simulink model "ansiBPF"  (R2018a)
settings: Solver=VariableStepAuto  StartTime=0.0  StopTime=0.001  RelTol=1e-3
undefined symbols (not defined in the file): fdesignblkfcn, G1, G10, G11, G12, G13, G14, G15, G16, G17, G18, G19, G2, G20, G21, G22, G23, G24, G25, G26, G3, G4, G5, G6, G7, G8, G9, gcbh, get, T
libraries: dspsrcs4 x1, dspxfrm3 x1, dspobslib x1
(part 2 of 8)

== system ansiBPF/Filter Bank /Filter 1/Bandpass Filter ==
  In : Inport
  Generated Filter Block : DiscreteFir  Tag=BlockMethodSubSystem  Coefficients=[0.0499507052705291318 0.000322270032915632448 0.000320188963324847956 0.000323977422964133151 0.000321713773073391111 0.000325363631786397078 0.000322903780407593076 0.000326435292404190028 0.000323726665637299603 0.000327135403143973057 0.000324164311384914105 0.000327508044235636268 0.000324274377688199664 0.000327562416867693297 0.000323957726949763232 0.000327232187704450399 0.000323344949635380897 0.000326624522215911107 0.000322307254760139392 0.00032580787553647487 0.000320960780481276359 0.000324697279934548508 0.000319257227297288124 0.000323532322174875826 0.000317320055412668978 0.000322525688887117048 0.000315188666134388798 0.000322272842734003641 0.000313133698767870767 0.000324938293286081007 0.000311846130644410772 0.000347911651016281258 0.000403441686760817907 0.000297983621868963587 0.000325553998969463972 0.000314801796637866754 0.000322376414307447051 0.000316225568461547747 0.000319627270835727822 0.000315367721629143639 0.000316827696566097548 0.000313550600974511317 0.000313841748774321551 0.000311178641818180696 0.000310645179700694935 0.000308339589890846433 0.000307082402857562927 0.00030506389195534921 0.000303289042348015166 0.000301392710367551664 0.000299107424724176681 0.000297449923396902593 0.000294574508449678548 0.000293085034438766946 0.000289703193611834018 0.000288524166281404896 0.000284574756131985857 0.000283864586364604053 0.000279247312497059091 0.00027950989385441366 0.000274059887801314614 0.000276778817366210507 0.000269800258802989237 0.000284929243345160492 0.000283667983013746879 0.000256341854324833524 0.000266246888784617503 0.000258441820358657945 0.000259919445659265625 0.000254271235270379003 0.000253863599798776569 0.000249074864716378533 0.000247701743744928619 0.000243346757243663713 0.00024135746450751195 0.000237267929251366465 0.000234794357897953599 0.00023080360466084252 0.000227870792300621783 0.000224002787101546024 0.000220716617566540094 0.000216796407569049151 0.000213204269357036554 0.000209323511238944897 0.000205277865080490173 0.000201412148869970322 0.000197030453623327732 0.000193257883064897366 0.000188493476993681667 0.000184903345259595614 0.000179758531360253672 0.00017669703079523582 0.0001712125296252561 0.000169594176652715855 0.000163669815242406888 0.000169209483617797527 0.000158691626351559895 0.000147141133803010521 0.000148689909581561111 0.000141419334482159468 0.000139026139903162128 0.000132817354956990422 0.000129471877618246014 0.000123647868192018444 0.000119769347168019225 0.000114128631332419424 0.000109899614122812946 0.000104355797795147015 9.98123926371075184e-05 9.42446037635563634e-05 8.94063108954827563e-05 8.38853496698552595e-05 7.87737989141462636e-05 7.31343128585705744e-05 6.78500081840607247e-05 6.21201361671771922e-05 5.64867904529115343e-05 5.07067815823427086e-05 4.48484184389351008e-05 3.9038446040410134e-05 3.29178180392793651e-05 2.71387403106747555e-05 2.08276072283989303e-05 1.53374637248327835e-05 8.9858584085083406e-06 4.34843225694638722e-06 -1.84041404762174528e-06 -2.61999962832273039e-06 -1.53795105204806869e-05 -2.23167825954521411e-05 -2.60238776460634881e-05 -3.35303089579822711e-05 -3.88675007855140896e-05 -4.59356687316810194e-05 -5.1714332151380571e-05 -5.86588787380864666e-05 -6.47087092550114023e-05 -7.15961180700431057e-05 -7.78259186883305221e-05 -8.47019799255221972e-05 -9.11297010712597624e-05 -9.80755165498401588e-05 -0.000104664659704481594 -0.000111595264430823393 -0.000118399687148734549 -0.000125440312275471613 -0.000132323624602139243 -0.000139529297481968365 -0.000146653678106061435 -0.000153918626685325337 -0.00016118239140813594 -0.000168535424938574872 -0.00017596314172899701 -0.000183348683518542473 -0.000190821075256901413 -0.000198039321408629101 -0.000205357267343941993 -0.00021208883464483543 -0.000218927092046725141 -0.000224088820977669527 -0.000236938143622294708 -0.000242792916361279367 -0.000249855402636313883 -0.000257730566739408781 -0.000265167623686717198 ...(+30966 chars)]  InputProcessing=Columns as channels (frame based)
  Out : Outport
  wires:
  In/1 -> Generated Filter Block/1
  Generated Filter Block/1 -> Out/1

== system ansiBPF/Filter Bank /Filter 10/Bandpass Filter ==
  In : Inport
  Generated Filter Block : DiscreteFir  Tag=BlockMethodSubSystem  Coefficients=[-0.00530401889529867176 -0.000762503662223860588 -0.000809597041362384662 -0.00085423713825715918 -0.000894486120251178156 -0.00093107548534541811 -0.000962288947070095253 -0.000989049435271363749 -0.00100934406038991867 -0.00102410104453707035 -0.00103149455372060885 -0.00103223687206899358 -0.00102448142749090036 -0.00100884844553548558 -0.000983515907192630172 -0.000949243642068295455 -0.000904319526077239279 -0.000849733841231411547 -0.000784037714204466958 -0.000708543736320957069 -0.000622127019485820172 -0.000526256294042048967 -0.000419644908513648965 -0.000303518853045686623 -0.000175943274000202999 -3.82552865238885645e-05 0.000111501683883899355 0.000270568478960216054 0.000438231571149218875 0.000609275407521666962 0.000787476786344833385 0.000986628487263300916 0.00117728994401449503 0.00137958302728576087 0.00158529722033642147 0.0017943167270931266 0.00200587609221354254 0.00221835053007343307 0.00243145506573108237 0.00264299880656624275 0.00285260919893783093 0.00305799897700812732 0.00325867434990166367 0.00345224276972189072 0.0036381525181242518 0.00381397827273103913 0.00397934470676978343 0.00413193515136546681 0.00427148440753266634 0.00439563199552642052 0.00450393141663923621 0.00459396169417253079 0.00466534335796109194 0.00471596849442543903 0.0047460829476344028 0.00475372894601983932 0.00473965666642539932 0.00470092950151681632 0.0046374213913586192 0.00454736880213954271 0.00443390292271470497 0.00429527524807777391 0.00412717617392089915 0.00393592745618333989 0.003717549896623055 0.00347337100296327616 0.00320396823719764842 0.00290931484653729911 0.00259092019299267135 0.00224862188594879839 0.00188446325206646933 0.00149863620390504608 0.00109346550765449489 0.000669391686506665292 0.00022891711714851542 -0.000227267110878131347 -0.000696281888405515911 -0.00117708989182640079 -0.00166649774040128159 -0.00216330051213994802 -0.00266433060412914636 -0.00316826631716930675 -0.00367190191018134608 -0.00417353296082717973 -0.00466960689996043232 -0.00515833134124038788 -0.00563589955200152586 -0.00610175871945096548 -0.00655196129802019904 -0.00698462243668052964 -0.00739547327021302433 -0.0077846372227648522 -0.00814879846851517507 -0.00848416723132251402 -0.00879058807074419371 -0.00906503847972718775 -0.00930543067975272975 -0.00951046410337792227 -0.00967774427538462163 -0.00980673524036465051 -0.00989502796839583469 -0.00994245078282056383 -0.00994696268261321265 -0.00990885487066216382 -0.00982662150586692019 -0.00970098126763126525 -0.00953077187132917066 -0.00931705690973690104 -0.00905904662331406124 -0.00875829750638353402 -0.00841465404343268338 -0.00803011316082513117 -0.0076051069870370679 -0.00714173367553548599 -0.00664085703672448978 -0.00610487290695389644 -0.00553514255694706123 -0.00493553731689033368 -0.00430658657183950657 -0.00365199467779552195 -0.00297358801683265646 -0.00227607748273341579 -0.00156041508850677472 -0.000830591097045980942 -9.02778463345356327e-05 0.000657701321223840181 0.00141012165207445592 0.00216301715968920906 0.00291355772225113541 0.00365735681289422162 0.00439198914739929048 0.00511302399646780363 0.00581814101116282911 0.00650291241124247802 0.00716505438872799393 0.0078003378917738328 0.00840677071557788605 0.00898045304128435376 0.00951971831009208735 0.0100209022066045667 0.0104825303066184029 0.0109013417773679965 0.0112761257041957674 0.0116044375129104368 0.0118852844436046212 0.012116974638974664 0.0122984597861088285 0.0124280462570238032 0.0125069270388523026 0.0125329151884100362 0.0125069270388523026 0.0124280462570238032 0.0122984597861088285 0.012116974638974664 0.0118852844436046212 0.0116044375129104368 0.0112761257041957674 0.0109013417773679965 0.0104825303066184029 0.0100209022066045667 0.00951971831009208735 0.00898045304128435376 0.00840677071557788605 0.0078003378917738328 0.00716505438872799393 0.00650291241124247802 0.00581814101116282911 0.00511302399646780363 0.00439198914739929048 0.00365735681289422162 ...(+3064 chars)]  InputProcessing=Columns as channels (frame based)
  Out : Outport
  wires:
  In/1 -> Generated Filter Block/1
  Generated Filter Block/1 -> Out/1
